simulink library "three_phase_inverter_three_level_ttype_igbt_based_model"  (R2026a)
settings: Solver=VariableStepAuto
undefined symbols (not defined in the file): DThs_init, glb_time, heatsink, igbt, Tambient
libraries: fl_lib x192, nesl_utility x108, ee_lib x24
(part 1 of 5)
settings Model: Creator=dbagn  LastModifiedBy=dbagn

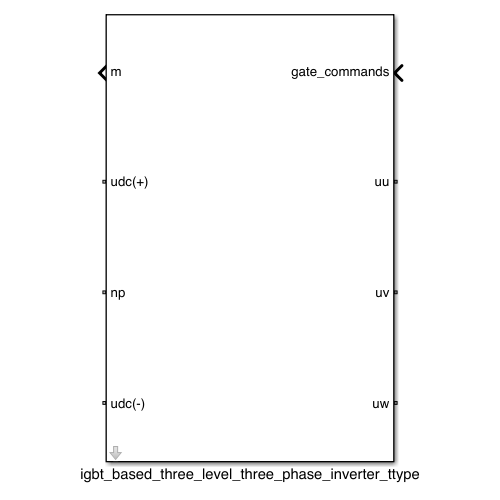
[thumbnail: Simulink's stored preview of the top-level diagram]
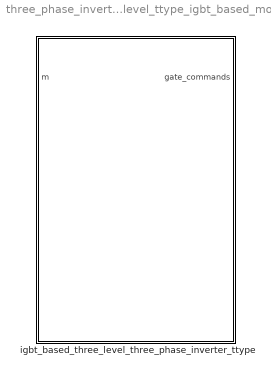
== system three_phase_inverter_three_level_ttype_igbt_based_model ==
  igbt_based_three_level_three_phase_inverter_ttype : Subsystem  mask{Vth_inv_t_m=igbt.afe.Vth, Vce_sat_inv_t_m=igbt.afe.Vce_sat, Rce_on_inv_t_m=igbt.afe.Rce_on, Eon_inv_t_m=igbt.afe.Eon, Eoff_inv_t_m=igbt.afe.Eoff, Erec_inv_t_m=igbt.afe.Erec, Ion_sw_loss_inv_t_m=igbt.afe.Ion_sw_losses, Voff_sw_loss_inv_t_m=igbt.afe.Voff_sw_losses, Vdon_diode_inv_t_m=igbt.afe.Vdon_diode, Rdon_diode_inv_t_m=igbt.afe.Rdon_diode, rth_switch_JH_inv_t_m=igbt.afe.Rth_switch_JH, rth_switch_HA_inv_t_m=heatsink.Rth_switch_HA, rth_diode_JH_inv_t_m=igbt.afe.Rth_diode_JH, rth_diode_HA_inv_t_m=heatsink.Rth_diode_HA, Csnubber_inv_t_m=igbt.afe.Csnubber, Rsnubber_inv_t_m=igbt.afe.Rsnubber, Vth_m=igbt.afe.Vth, Vce_sat_m=igbt.afe.Vce_sat, Rce_on_m=igbt.afe.Rce_on, Eon_m=igbt.afe.Eon, Eoff_m=igbt.afe.Eoff, Erec_m=igbt.afe.Erec, Ion_sw_loss_m=igbt.afe.Ion_sw_losses, Voff_sw_loss_m=igbt.afe.Voff_sw_losses, Vdon_diode_m=igbt.afe.Vdon_diode, Rdon_diode_m=igbt.afe.Rdon_diode, rth_switch_JH_m=igbt.afe.Rth_switch_JH, rth_switch_HA_m=heatsink.Rth_switch_HA, rth_diode_JH_m=igbt.afe.Rth_diode_JH, rth_diode_HA_m=heatsink.Rth_diode_HA, Csnubber_m=igbt.afe.Csnubber, Rsnubber_m=igbt.afe.Rsnubber, JunctionTermalMass_m=igbt.afe.JunctionTermalMass, mass_heatsink_m=heatsink.no_weight, specific_heat_m=heatsink.cp, Tambient_m=heatsink.Tambient, DThs_init_m=heatsink.DThs_init, tc_m=glb_time.tc}
      mask prompts: Vth_inv_t_m "Vth (V)"; Vce_sat_inv_t_m "Vce_sat (V)"; Rce_on_inv_t_m "Rce_on (Ohm)"; Eon_inv_t_m "Eon (J)"; Eoff_inv_t_m "Eoff (J)"; Erec_inv_t_m "Erec (J)"; Ion_sw_loss_inv_t_m "Ion_sw_loss (A)"; Voff_sw_loss_inv_t_m "Voff_sw_loss (V)"; Vdon_diode_inv_t_m "Vdon_diode (V)"; Rdon_diode_inv_t_m "Rdon_diode (Ohm)"; rth_switch_JH_inv_t_m "rth_switch_JH (K/W)"; rth_switch_HA_inv_t_m "rth_switch_HA  (K/W)"; rth_diode_JH_inv_t_m "rth_diode_JH (K/W)"; rth_diode_HA_inv_t_m "rth_diode_HA  (K/W)"; Csnubber_inv_t_m "Csnubber (F)"; Rsnubber_inv_t_m "Rsnubber (Ohm)"; Vth_m "Vth (V)"; Vce_sat_m "Vce_sat (V)"; Rce_on_m "Rce_on (Ohm)"; Eon_m "Eon (J)"; Eoff_m "Eoff (J)"; Erec_m "Erec (J)"; Ion_sw_loss_m "Ion_sw_loss (A)"; Voff_sw_loss_m "Voff_sw_loss (V)"; Vdon_diode_m "Vdon_diode (V)"; Rdon_diode_m "Rdon_diode (Ohm)"; rth_switch_JH_m "rth_switch_JH (K/W)"; rth_switch_HA_m "rth_switch_HA  (K/W)"; rth_diode_JH_m "rth_diode_JH (K/W)"; rth_diode_HA_m "rth_diode_HA  (K/W)"; Csnubber_m "Csnubber (F)"; Rsnubber_m "Rsnubber (Ohm)"; JunctionTermalMass_m "JunctionTermalMass (J/K)"; mass_heatsink_m "mass_heatsink (Kg)"; specific_heat_m "specific_heat (J/(K*Kg))"; Tambient_m "Tambient (Celsius)"; DThs_init_m "DThs_init (Celsius)"; tc_m "tc"
      mask DialogControl inv_t Prompt: T-IGBT
      mask DialogControl inv Prompt: IGBT
      mask DialogControl thermal Prompt: Thermal
      mask DialogControl solver Prompt: Solver

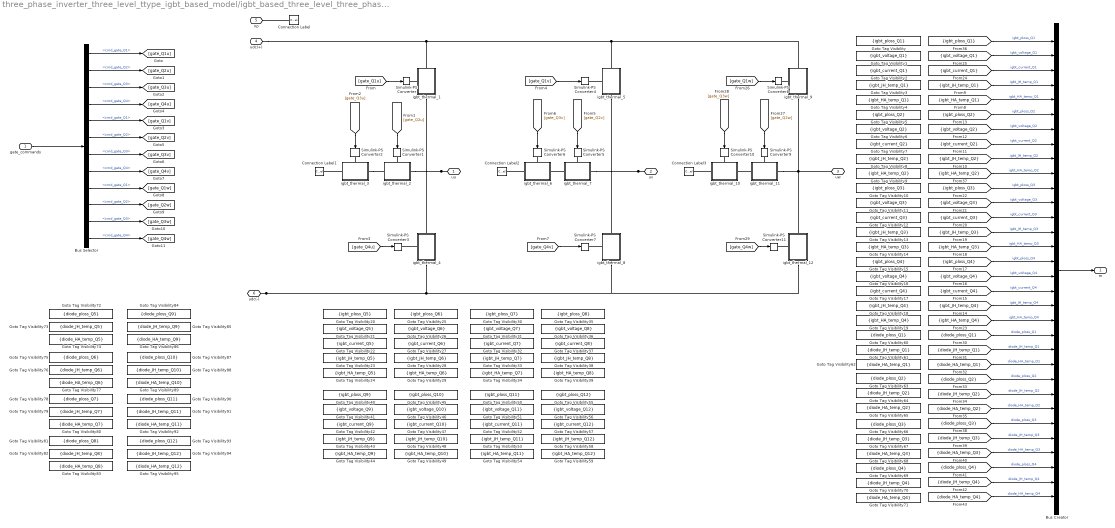
== system three_phase_inverter_three_level_ttype_igbt_based_model/igbt_based_three_level_three_phase_inverter_ttype ==
  gate_commands : Inport
  Bus Creator : BusCreator  Inputs=32
  Bus Selector : BusSelector  OutputSignals=gate_cmds_phu.cmd_gate_Q1,gate_cmds_phu.cmd_gate_Q2,gate_cmds_phu.cmd_gate_Q3,gate_cmds_phu.cmd_gate_Q4,gate_cmds_phv.cmd_gate_Q1,gate_cmds_phv.cmd_gate_Q2,gate_cmds_phv.cmd_gate_Q3,gate_cmds_phv.cmd_gate_Q4,gate_cmds_phw.cmd_gate_Q1,gate_cmds_phw.cmd_gate_Q2,gate_cmds_phw.cmd_gate_Q3,gate_cmds_phw.cmd_gate_Q4
  Connection Label{,1..3} (4 alike) : ConnectionLabel  Label=np
  Goto Tag Visibility : GotoTagVisibility  GotoTag=igbt_ploss_Q1
  Goto Tag Visibility1 : GotoTagVisibility  GotoTag=igbt_voltage_Q1
  Goto Tag Visibility10 : GotoTagVisibility  GotoTag=igbt_ploss_Q3
  Goto Tag Visibility11 : GotoTagVisibility  GotoTag=igbt_voltage_Q3
  Goto Tag Visibility12 : GotoTagVisibility  GotoTag=igbt_current_Q3
  Goto Tag Visibility13 : GotoTagVisibility  GotoTag=igbt_JH_temp_Q3
  Goto Tag Visibility14 : GotoTagVisibility  GotoTag=igbt_HA_temp_Q3
  Goto Tag Visibility15 : GotoTagVisibility  GotoTag=igbt_ploss_Q4
  Goto Tag Visibility16 : GotoTagVisibility  GotoTag=igbt_voltage_Q4
  Goto Tag Visibility17 : GotoTagVisibility  GotoTag=igbt_current_Q4
  Goto Tag Visibility18 : GotoTagVisibility  GotoTag=igbt_JH_temp_Q4
  Goto Tag Visibility19 : GotoTagVisibility  GotoTag=igbt_HA_temp_Q4
  Goto Tag Visibility2 : GotoTagVisibility  GotoTag=igbt_current_Q1
  Goto Tag Visibility20 : GotoTagVisibility  GotoTag=igbt_ploss_Q5
  Goto Tag Visibility21 : GotoTagVisibility  GotoTag=igbt_voltage_Q5
  Goto Tag Visibility22 : GotoTagVisibility  GotoTag=igbt_current_Q5
  Goto Tag Visibility23 : GotoTagVisibility  GotoTag=igbt_JH_temp_Q5
  Goto Tag Visibility24 : GotoTagVisibility  GotoTag=igbt_HA_temp_Q5
  Goto Tag Visibility25 : GotoTagVisibility  GotoTag=igbt_ploss_Q6
  Goto Tag Visibility26 : GotoTagVisibility  GotoTag=igbt_voltage_Q6
  Goto Tag Visibility27 : GotoTagVisibility  GotoTag=igbt_current_Q6
  Goto Tag Visibility28 : GotoTagVisibility  GotoTag=igbt_JH_temp_Q6
  Goto Tag Visibility29 : GotoTagVisibility  GotoTag=igbt_HA_temp_Q6
  Goto Tag Visibility3 : GotoTagVisibility  GotoTag=igbt_JH_temp_Q1
  Goto Tag Visibility30 : GotoTagVisibility  GotoTag=igbt_ploss_Q7
  Goto Tag Visibility31 : GotoTagVisibility  GotoTag=igbt_voltage_Q7
  Goto Tag Visibility32 : GotoTagVisibility  GotoTag=igbt_current_Q7
  Goto Tag Visibility33 : GotoTagVisibility  GotoTag=igbt_JH_temp_Q7
  Goto Tag Visibility34 : GotoTagVisibility  GotoTag=igbt_HA_temp_Q7
  Goto Tag Visibility35 : GotoTagVisibility  GotoTag=igbt_ploss_Q8
  Goto Tag Visibility36 : GotoTagVisibility  GotoTag=igbt_voltage_Q8
  Goto Tag Visibility37 : GotoTagVisibility  GotoTag=igbt_current_Q8
  Goto Tag Visibility38 : GotoTagVisibility  GotoTag=igbt_JH_temp_Q8
  Goto Tag Visibility39 : GotoTagVisibility  GotoTag=igbt_HA_temp_Q8
  Goto Tag Visibility4 : GotoTagVisibility  GotoTag=igbt_HA_temp_Q1
  Goto Tag Visibility40 : GotoTagVisibility  GotoTag=igbt_ploss_Q9
  Goto Tag Visibility41 : GotoTagVisibility  GotoTag=igbt_voltage_Q9
  Goto Tag Visibility42 : GotoTagVisibility  GotoTag=igbt_current_Q9
  Goto Tag Visibility43 : GotoTagVisibility  GotoTag=igbt_JH_temp_Q9
  Goto Tag Visibility44 : GotoTagVisibility  GotoTag=igbt_HA_temp_Q9
  Goto Tag Visibility45 : GotoTagVisibility  GotoTag=igbt_ploss_Q10
  Goto Tag Visibility46 : GotoTagVisibility  GotoTag=igbt_voltage_Q10
  Goto Tag Visibility47 : GotoTagVisibility  GotoTag=igbt_current_Q10
  Goto Tag Visibility48 : GotoTagVisibility  GotoTag=igbt_JH_temp_Q10
  Goto Tag Visibility49 : GotoTagVisibility  GotoTag=igbt_HA_temp_Q10
  Goto Tag Visibility5 : GotoTagVisibility  GotoTag=igbt_ploss_Q2
  Goto Tag Visibility50 : GotoTagVisibility  GotoTag=igbt_ploss_Q11
  Goto Tag Visibility51 : GotoTagVisibility  GotoTag=igbt_voltage_Q11
  Goto Tag Visibility52 : GotoTagVisibility  GotoTag=igbt_current_Q11
  Goto Tag Visibility53 : GotoTagVisibility  GotoTag=igbt_JH_temp_Q11
  Goto Tag Visibility54 : GotoTagVisibility  GotoTag=igbt_HA_temp_Q11
  Goto Tag Visibility55 : GotoTagVisibility  GotoTag=igbt_ploss_Q12
  Goto Tag Visibility56 : GotoTagVisibility  GotoTag=igbt_voltage_Q12
  Goto Tag Visibility57 : GotoTagVisibility  GotoTag=igbt_current_Q12
  Goto Tag Visibility58 : GotoTagVisibility  GotoTag=igbt_JH_temp_Q12
  Goto Tag Visibility59 : GotoTagVisibility  GotoTag=igbt_HA_temp_Q12
  Goto Tag Visibility6 : GotoTagVisibility  GotoTag=igbt_voltage_Q2
  Goto Tag Visibility60 : GotoTagVisibility  GotoTag=diode_ploss_Q1
  Goto Tag Visibility61 : GotoTagVisibility  GotoTag=diode_JH_temp_Q1
  Goto Tag Visibility62 : GotoTagVisibility  GotoTag=diode_HA_temp_Q1
  Goto Tag Visibility63 : GotoTagVisibility  GotoTag=diode_ploss_Q2
  Goto Tag Visibility64 : GotoTagVisibility  GotoTag=diode_JH_temp_Q2
  Goto Tag Visibility65 : GotoTagVisibility  GotoTag=diode_HA_temp_Q2
  Goto Tag Visibility66 : GotoTagVisibility  GotoTag=diode_ploss_Q3
  Goto Tag Visibility67 : GotoTagVisibility  GotoTag=diode_JH_temp_Q3
  Goto Tag Visibility68 : GotoTagVisibility  GotoTag=diode_HA_temp_Q3
  Goto Tag Visibility69 : GotoTagVisibility  GotoTag=diode_ploss_Q4
  Goto Tag Visibility7 : GotoTagVisibility  GotoTag=igbt_current_Q2
  Goto Tag Visibility70 : GotoTagVisibility  GotoTag=diode_JH_temp_Q4
  Goto Tag Visibility71 : GotoTagVisibility  GotoTag=diode_HA_temp_Q4
  Goto Tag Visibility72 : GotoTagVisibility  GotoTag=diode_ploss_Q5
  Goto Tag Visibility73 : GotoTagVisibility  GotoTag=diode_JH_temp_Q5
  Goto Tag Visibility74 : GotoTagVisibility  GotoTag=diode_HA_temp_Q5
  Goto Tag Visibility75 : GotoTagVisibility  GotoTag=diode_ploss_Q6
  Goto Tag Visibility76 : GotoTagVisibility  GotoTag=diode_JH_temp_Q6
  Goto Tag Visibility77 : GotoTagVisibility  GotoTag=diode_HA_temp_Q6
  Goto Tag Visibility78 : GotoTagVisibility  GotoTag=diode_ploss_Q7
  Goto Tag Visibility79 : GotoTagVisibility  GotoTag=diode_JH_temp_Q7
  Goto Tag Visibility8 : GotoTagVisibility  GotoTag=igbt_JH_temp_Q2
  Goto Tag Visibility80 : GotoTagVisibility  GotoTag=diode_HA_temp_Q7
  Goto Tag Visibility81 : GotoTagVisibility  GotoTag=diode_ploss_Q8
  Goto Tag Visibility82 : GotoTagVisibility  GotoTag=diode_JH_temp_Q8
  Goto Tag Visibility83 : GotoTagVisibility  GotoTag=diode_HA_temp_Q8
  Goto Tag Visibility84 : GotoTagVisibility  GotoTag=diode_ploss_Q9
  Goto Tag Visibility85 : GotoTagVisibility  GotoTag=diode_JH_temp_Q9
  Goto Tag Visibility86 : GotoTagVisibility  GotoTag=diode_HA_temp_Q9
  Goto Tag Visibility87 : GotoTagVisibility  GotoTag=diode_ploss_Q10
  Goto Tag Visibility88 : GotoTagVisibility  GotoTag=diode_JH_temp_Q10
  Goto Tag Visibility89 : GotoTagVisibility  GotoTag=diode_HA_temp_Q10
  Goto Tag Visibility9 : GotoTagVisibility  GotoTag=igbt_HA_temp_Q2
  Goto Tag Visibility90 : GotoTagVisibility  GotoTag=diode_ploss_Q11
  Goto Tag Visibility91 : GotoTagVisibility  GotoTag=diode_JH_temp_Q11
  Goto Tag Visibility92 : GotoTagVisibility  GotoTag=diode_HA_temp_Q11
  Goto Tag Visibility93 : GotoTagVisibility  GotoTag=diode_ploss_Q12
  Goto Tag Visibility94 : GotoTagVisibility  GotoTag=diode_JH_temp_Q12
  Goto Tag Visibility95 : GotoTagVisibility  GotoTag=diode_HA_temp_Q12
  Simulink-PS Converter{,1..11} (12 alike) : nesl_utility/Simulink-PS Converter  PhysicalDomain=network_engine_domain  SubClassName=ps_input  LeftPortType=input  RightPortType=output  PseudoPeriodic=off  Frequencies=[]  NoiseDistribution=none  NoiseParameters=[]  Unit=1  AffineConversion=on  FilteringAndDerivatives=provide  SimscapeFilterOrder=1  InputFilterTimeConstant=0.001  UdotUserProvided=0
  igbt_thermal_1 : Subsystem
      settings: PortSchema="{\"entries\":[{\"content\":{\"sides\":[{\"content\":{\"connectorIds\":[\"LConn1\"]},\"type\":\"ConnectorPlacement.EquallySpacedRectSide\",\"uuid\":\"9277da8d-d460-43e6-8478-dd662f15d226\"},{\"content\":{\"connectorIds\":[],\"side\":\"RIGHT\"},\"type\":\"ConnectorPlacement.EquallySpacedRectSide\",\"uuid\":\"a7ece396-f1d9-4f4f-a05b-db1fc65d6e1d\"},{\"content\":{\"connectorIds\":[\"LConn2\"],\"side\":\"TOP\"},\"type\":\"ConnectorPlacement.EquallySpacedRectSide\",\"uuid\":\"fdd70777-e9cf-4317-afb6-cae87f75d5b0\"},{\"content\":{\"connectorIds\":[\"RConn1\"],\"side\":\"BOTTOM\"},\"type\":\"ConnectorPlacement.EquallySpacedRectSide\",\"uuid\":\"2353ed68-b1a1-4775-9ca9-31e268d5443b\"}]},\"type\":\"ConnectorPlacement.EquallySpacedConnector\",\"uuid\":\"d5479f4c-4e65-4791-adcb-73df11f88590\"}],\"packageUris\":[\"http://schema.mathworks.com/mf0/Connector/R2020b\"],\"version\":\"1.0\"}"
  igbt_thermal_10 : Subsystem
      settings: PortSchema="{\"entries\":[{\"content\":{\"sides\":[{\"content\":{\"connectorIds\":[\"LConn1\"]},\"type\":\"ConnectorPlacement.EquallySpacedRectSide\",\"uuid\":\"9277da8d-d460-43e6-8478-dd662f15d226\"},{\"content\":{\"connectorIds\":[],\"side\":\"RIGHT\"},\"type\":\"ConnectorPlacement.EquallySpacedRectSide\",\"uuid\":\"a7ece396-f1d9-4f4f-a05b-db1fc65d6e1d\"},{\"content\":{\"connectorIds\":[\"LConn2\"],\"side\":\"TOP\"},\"type\":\"ConnectorPlacement.EquallySpacedRectSide\",\"uuid\":\"fdd70777-e9cf-4317-afb6-cae87f75d5b0\"},{\"content\":{\"connectorIds\":[\"RConn1\"],\"side\":\"BOTTOM\"},\"type\":\"ConnectorPlacement.EquallySpacedRectSide\",\"uuid\":\"2353ed68-b1a1-4775-9ca9-31e268d5443b\"}]},\"type\":\"ConnectorPlacement.EquallySpacedConnector\",\"uuid\":\"d5479f4c-4e65-4791-adcb-73df11f88590\"}],\"packageUris\":[\"http://schema.mathworks.com/mf0/Connector/R2020b\"],\"version\":\"1.0\"}"
  igbt_thermal_11 : Subsystem
      settings: PortSchema="{\"entries\":[{\"content\":{\"sides\":[{\"content\":{\"connectorIds\":[\"LConn1\"]},\"type\":\"ConnectorPlacement.EquallySpacedRectSide\",\"uuid\":\"9277da8d-d460-43e6-8478-dd662f15d226\"},{\"content\":{\"connectorIds\":[],\"side\":\"RIGHT\"},\"type\":\"ConnectorPlacement.EquallySpacedRectSide\",\"uuid\":\"a7ece396-f1d9-4f4f-a05b-db1fc65d6e1d\"},{\"content\":{\"connectorIds\":[\"LConn2\"],\"side\":\"TOP\"},\"type\":\"ConnectorPlacement.EquallySpacedRectSide\",\"uuid\":\"fdd70777-e9cf-4317-afb6-cae87f75d5b0\"},{\"content\":{\"connectorIds\":[\"RConn1\"],\"side\":\"BOTTOM\"},\"type\":\"ConnectorPlacement.EquallySpacedRectSide\",\"uuid\":\"2353ed68-b1a1-4775-9ca9-31e268d5443b\"}]},\"type\":\"ConnectorPlacement.EquallySpacedConnector\",\"uuid\":\"d5479f4c-4e65-4791-adcb-73df11f88590\"}],\"packageUris\":[\"http://schema.mathworks.com/mf0/Connector/R2020b\"],\"version\":\"1.0\"}"
  igbt_thermal_12 : Subsystem
      settings: PortSchema="{\"entries\":[{\"content\":{\"sides\":[{\"content\":{\"connectorIds\":[\"LConn1\"]},\"type\":\"ConnectorPlacement.EquallySpacedRectSide\",\"uuid\":\"9277da8d-d460-43e6-8478-dd662f15d226\"},{\"content\":{\"connectorIds\":[],\"side\":\"RIGHT\"},\"type\":\"ConnectorPlacement.EquallySpacedRectSide\",\"uuid\":\"a7ece396-f1d9-4f4f-a05b-db1fc65d6e1d\"},{\"content\":{\"connectorIds\":[\"LConn2\"],\"side\":\"TOP\"},\"type\":\"ConnectorPlacement.EquallySpacedRectSide\",\"uuid\":\"fdd70777-e9cf-4317-afb6-cae87f75d5b0\"},{\"content\":{\"connectorIds\":[\"RConn1\"],\"side\":\"BOTTOM\"},\"type\":\"ConnectorPlacement.EquallySpacedRectSide\",\"uuid\":\"2353ed68-b1a1-4775-9ca9-31e268d5443b\"}]},\"type\":\"ConnectorPlacement.EquallySpacedConnector\",\"uuid\":\"d5479f4c-4e65-4791-adcb-73df11f88590\"}],\"packageUris\":[\"http://schema.mathworks.com/mf0/Connector/R2020b\"],\"version\":\"1.0\"}"
  igbt_thermal_2 : Subsystem
      settings: PortSchema="{\"entries\":[{\"content\":{\"sides\":[{\"content\":{\"connectorIds\":[\"LConn1\"]},\"type\":\"ConnectorPlacement.EquallySpacedRectSide\",\"uuid\":\"9277da8d-d460-43e6-8478-dd662f15d226\"},{\"content\":{\"connectorIds\":[],\"side\":\"RIGHT\"},\"type\":\"ConnectorPlacement.EquallySpacedRectSide\",\"uuid\":\"a7ece396-f1d9-4f4f-a05b-db1fc65d6e1d\"},{\"content\":{\"connectorIds\":[\"LConn2\"],\"side\":\"TOP\"},\"type\":\"ConnectorPlacement.EquallySpacedRectSide\",\"uuid\":\"fdd70777-e9cf-4317-afb6-cae87f75d5b0\"},{\"content\":{\"connectorIds\":[\"RConn1\"],\"side\":\"BOTTOM\"},\"type\":\"ConnectorPlacement.EquallySpacedRectSide\",\"uuid\":\"2353ed68-b1a1-4775-9ca9-31e268d5443b\"}]},\"type\":\"ConnectorPlacement.EquallySpacedConnector\",\"uuid\":\"d5479f4c-4e65-4791-adcb-73df11f88590\"}],\"packageUris\":[\"http://schema.mathworks.com/mf0/Connector/R2020b\"],\"version\":\"1.0\"}"
  igbt_thermal_3 : Subsystem
      settings: PortSchema="{\"entries\":[{\"content\":{\"sides\":[{\"content\":{\"connectorIds\":[\"LConn1\"]},\"type\":\"ConnectorPlacement.EquallySpacedRectSide\",\"uuid\":\"9277da8d-d460-43e6-8478-dd662f15d226\"},{\"content\":{\"side\":\"RIGHT\"},\"type\":\"ConnectorPlacement.EquallySpacedRectSide\",\"uuid\":\"a7ece396-f1d9-4f4f-a05b-db1fc65d6e1d\"},{\"content\":{\"connectorIds\":[\"LConn2\"],\"side\":\"TOP\"},\"type\":\"ConnectorPlacement.EquallySpacedRectSide\",\"uuid\":\"fdd70777-e9cf-4317-afb6-cae87f75d5b0\"},{\"content\":{\"connectorIds\":[\"RConn1\"],\"side\":\"BOTTOM\"},\"type\":\"ConnectorPlacement.EquallySpacedRectSide\",\"uuid\":\"2353ed68-b1a1-4775-9ca9-31e268d5443b\"}]},\"type\":\"ConnectorPlacement.EquallySpacedConnector\",\"uuid\":\"d5479f4c-4e65-4791-adcb-73df11f88590\"}],\"packageUris\":[\"http://schema.mathworks.com/mf0/Connector/R2020b\"],\"version\":\"1.0\"}"
  igbt_thermal_4 : Subsystem
      settings: PortSchema="{\"entries\":[{\"content\":{\"sides\":[{\"content\":{\"connectorIds\":[\"LConn1\"]},\"type\":\"ConnectorPlacement.EquallySpacedRectSide\",\"uuid\":\"9277da8d-d460-43e6-8478-dd662f15d226\"},{\"content\":{\"connectorIds\":[],\"side\":\"RIGHT\"},\"type\":\"ConnectorPlacement.EquallySpacedRectSide\",\"uuid\":\"a7ece396-f1d9-4f4f-a05b-db1fc65d6e1d\"},{\"content\":{\"connectorIds\":[\"LConn2\"],\"side\":\"TOP\"},\"type\":\"ConnectorPlacement.EquallySpacedRectSide\",\"uuid\":\"fdd70777-e9cf-4317-afb6-cae87f75d5b0\"},{\"content\":{\"connectorIds\":[\"RConn1\"],\"side\":\"BOTTOM\"},\"type\":\"ConnectorPlacement.EquallySpacedRectSide\",\"uuid\":\"2353ed68-b1a1-4775-9ca9-31e268d5443b\"}]},\"type\":\"ConnectorPlacement.EquallySpacedConnector\",\"uuid\":\"d5479f4c-4e65-4791-adcb-73df11f88590\"}],\"packageUris\":[\"http://schema.mathworks.com/mf0/Connector/R2020b\"],\"version\":\"1.0\"}"
  igbt_thermal_5 : Subsystem
      settings: PortSchema="{\"entries\":[{\"content\":{\"sides\":[{\"content\":{\"connectorIds\":[\"LConn1\"]},\"type\":\"ConnectorPlacement.EquallySpacedRectSide\",\"uuid\":\"9277da8d-d460-43e6-8478-dd662f15d226\"},{\"content\":{\"connectorIds\":[],\"side\":\"RIGHT\"},\"type\":\"ConnectorPlacement.EquallySpacedRectSide\",\"uuid\":\"a7ece396-f1d9-4f4f-a05b-db1fc65d6e1d\"},{\"content\":{\"connectorIds\":[\"LConn2\"],\"side\":\"TOP\"},\"type\":\"ConnectorPlacement.EquallySpacedRectSide\",\"uuid\":\"fdd70777-e9cf-4317-afb6-cae87f75d5b0\"},{\"content\":{\"connectorIds\":[\"RConn1\"],\"side\":\"BOTTOM\"},\"type\":\"ConnectorPlacement.EquallySpacedRectSide\",\"uuid\":\"2353ed68-b1a1-4775-9ca9-31e268d5443b\"}]},\"type\":\"ConnectorPlacement.EquallySpacedConnector\",\"uuid\":\"d5479f4c-4e65-4791-adcb-73df11f88590\"}],\"packageUris\":[\"http://schema.mathworks.com/mf0/Connector/R2020b\"],\"version\":\"1.0\"}"
  igbt_thermal_6 : Subsystem
      settings: PortSchema="{\"entries\":[{\"content\":{\"sides\":[{\"content\":{\"connectorIds\":[\"LConn1\"]},\"type\":\"ConnectorPlacement.EquallySpacedRectSide\",\"uuid\":\"9277da8d-d460-43e6-8478-dd662f15d226\"},{\"content\":{\"side\":\"RIGHT\"},\"type\":\"ConnectorPlacement.EquallySpacedRectSide\",\"uuid\":\"a7ece396-f1d9-4f4f-a05b-db1fc65d6e1d\"},{\"content\":{\"connectorIds\":[\"LConn2\"],\"side\":\"TOP\"},\"type\":\"ConnectorPlacement.EquallySpacedRectSide\",\"uuid\":\"fdd70777-e9cf-4317-afb6-cae87f75d5b0\"},{\"content\":{\"connectorIds\":[\"RConn1\"],\"side\":\"BOTTOM\"},\"type\":\"ConnectorPlacement.EquallySpacedRectSide\",\"uuid\":\"2353ed68-b1a1-4775-9ca9-31e268d5443b\"}]},\"type\":\"ConnectorPlacement.EquallySpacedConnector\",\"uuid\":\"d5479f4c-4e65-4791-adcb-73df11f88590\"}],\"packageUris\":[\"http://schema.mathworks.com/mf0/Connector/R2020b\"],\"version\":\"1.0\"}"
  igbt_thermal_7 : Subsystem
      settings: PortSchema="{\"entries\":[{\"content\":{\"sides\":[{\"content\":{\"connectorIds\":[\"LConn1\"]},\"type\":\"ConnectorPlacement.EquallySpacedRectSide\",\"uuid\":\"9277da8d-d460-43e6-8478-dd662f15d226\"},{\"content\":{\"connectorIds\":[],\"side\":\"RIGHT\"},\"type\":\"ConnectorPlacement.EquallySpacedRectSide\",\"uuid\":\"a7ece396-f1d9-4f4f-a05b-db1fc65d6e1d\"},{\"content\":{\"connectorIds\":[\"LConn2\"],\"side\":\"TOP\"},\"type\":\"ConnectorPlacement.EquallySpacedRectSide\",\"uuid\":\"fdd70777-e9cf-4317-afb6-cae87f75d5b0\"},{\"content\":{\"connectorIds\":[\"RConn1\"],\"side\":\"BOTTOM\"},\"type\":\"ConnectorPlacement.EquallySpacedRectSide\",\"uuid\":\"2353ed68-b1a1-4775-9ca9-31e268d5443b\"}]},\"type\":\"ConnectorPlacement.EquallySpacedConnector\",\"uuid\":\"d5479f4c-4e65-4791-adcb-73df11f88590\"}],\"packageUris\":[\"http://schema.mathworks.com/mf0/Connector/R2020b\"],\"version\":\"1.0\"}"
  igbt_thermal_8 : Subsystem
      settings: PortSchema="{\"entries\":[{\"content\":{\"sides\":[{\"content\":{\"connectorIds\":[\"LConn1\"]},\"type\":\"ConnectorPlacement.EquallySpacedRectSide\",\"uuid\":\"9277da8d-d460-43e6-8478-dd662f15d226\"},{\"content\":{\"connectorIds\":[],\"side\":\"RIGHT\"},\"type\":\"ConnectorPlacement.EquallySpacedRectSide\",\"uuid\":\"a7ece396-f1d9-4f4f-a05b-db1fc65d6e1d\"},{\"content\":{\"connectorIds\":[\"LConn2\"],\"side\":\"TOP\"},\"type\":\"ConnectorPlacement.EquallySpacedRectSide\",\"uuid\":\"fdd70777-e9cf-4317-afb6-cae87f75d5b0\"},{\"content\":{\"connectorIds\":[\"RConn1\"],\"side\":\"BOTTOM\"},\"type\":\"ConnectorPlacement.EquallySpacedRectSide\",\"uuid\":\"2353ed68-b1a1-4775-9ca9-31e268d5443b\"}]},\"type\":\"ConnectorPlacement.EquallySpacedConnector\",\"uuid\":\"d5479f4c-4e65-4791-adcb-73df11f88590\"}],\"packageUris\":[\"http://schema.mathworks.com/mf0/Connector/R2020b\"],\"version\":\"1.0\"}"
  igbt_thermal_9 : Subsystem
      settings: PortSchema="{\"entries\":[{\"content\":{\"sides\":[{\"content\":{\"connectorIds\":[\"LConn1\"]},\"type\":\"ConnectorPlacement.EquallySpacedRectSide\",\"uuid\":\"9277da8d-d460-43e6-8478-dd662f15d226\"},{\"content\":{\"connectorIds\":[],\"side\":\"RIGHT\"},\"type\":\"ConnectorPlacement.EquallySpacedRectSide\",\"uuid\":\"a7ece396-f1d9-4f4f-a05b-db1fc65d6e1d\"},{\"content\":{\"connectorIds\":[\"LConn2\"],\"side\":\"TOP\"},\"type\":\"ConnectorPlacement.EquallySpacedRectSide\",\"uuid\":\"fdd70777-e9cf-4317-afb6-cae87f75d5b0\"},{\"content\":{\"connectorIds\":[\"RConn1\"],\"side\":\"BOTTOM\"},\"type\":\"ConnectorPlacement.EquallySpacedRectSide\",\"uuid\":\"2353ed68-b1a1-4775-9ca9-31e268d5443b\"}]},\"type\":\"ConnectorPlacement.EquallySpacedConnector\",\"uuid\":\"d5479f4c-4e65-4791-adcb-73df11f88590\"}],\"packageUris\":[\"http://schema.mathworks.com/mf0/Connector/R2020b\"],\"version\":\"1.0\"}"
  uu : PMIOPort  Side=Left
  uv : PMIOPort  Port=2  Side=Left
  uw : PMIOPort  Port=3  Side=Left
  udc(+) : PMIOPort  Port=4  Side=Right
  np : PMIOPort  Port=5  Side=Right
  udc(-) : PMIOPort  Port=6  Side=Right
  m : Outport
  wires:
  [gate_Q4u] -> Simulink-PS Converter3/1
  [gate_Q3u] -> Simulink-PS Converter2/1
  [gate_Q2u] -> Simulink-PS Converter1/1
  [gate_Q1u] -> Simulink-PS Converter/1
  [gate_Q1v] -> Simulink-PS Converter4/1
  [gate_Q2v] -> Simulink-PS Converter5/1
  [gate_Q3v] -> Simulink-PS Converter6/1
  [gate_Q4v] -> Simulink-PS Converter7/1
  gate_commands/1 -> Bus Selector/1
  [igbt_voltage_Q1] -> Bus Creator/2  "igbt_voltage_Q1"
  [igbt_current_Q4] -> Bus Creator/18  "igbt_current_Q4"
  [igbt_voltage_Q2] -> Bus Creator/7  "igbt_voltage_Q2"
  [igbt_ploss_Q2] -> Bus Creator/6  "igbt_ploss_Q2"
  Bus Creator/1 -> m/1
  [igbt_ploss_Q3] -> Bus Creator/11  "igbt_ploss_Q3"
  [igbt_HA_temp_Q1] -> Bus Creator/5  "igbt_HA_temp_Q1"
  [igbt_ploss_Q1] -> Bus Creator/1  "igbt_ploss_Q1"
  [igbt_voltage_Q4] -> Bus Creator/17  "igbt_voltage_Q4"
  [igbt_ploss_Q4] -> Bus Creator/16  "igbt_ploss_Q4"
  [igbt_JH_temp_Q4] -> Bus Creator/19  "igbt_JH_temp_Q4"
  [igbt_voltage_Q3] -> Bus Creator/12  "igbt_voltage_Q3"
  [igbt_current_Q1] -> Bus Creator/3  "igbt_current_Q1"
  [igbt_HA_temp_Q4] -> Bus Creator/20  "igbt_HA_temp_Q4"
  [igbt_JH_temp_Q3] -> Bus Creator/14  "igbt_JH_temp_Q3"
  [igbt_current_Q2] -> Bus Creator/8  "igbt_current_Q2"
  [igbt_HA_temp_Q2] -> Bus Creator/10  "igbt_HA_temp_Q2"
  [igbt_JH_temp_Q2] -> Bus Creator/9  "igbt_JH_temp_Q2"
  [igbt_JH_temp_Q1] -> Bus Creator/4  "igbt_JH_temp_Q1"
  [igbt_current_Q3] -> Bus Creator/13  "igbt_current_Q3"
  [igbt_HA_temp_Q3] -> Bus Creator/15  "igbt_HA_temp_Q3"
  [gate_Q4w] -> Simulink-PS Converter11/1
  [gate_Q3w] -> Simulink-PS Converter10/1
  [gate_Q2w] -> Simulink-PS Converter9/1
  [gate_Q1w] -> Simulink-PS Converter8/1
  [diode_ploss_Q1] -> Bus Creator/21  "diode_ploss_Q1"
  [diode_JH_temp_Q1] -> Bus Creator/22  "diode_JH_temp_Q1"
  [diode_HA_temp_Q1] -> Bus Creator/23  "diode_HA_temp_Q1"
  [diode_ploss_Q2] -> Bus Creator/24  "diode_ploss_Q2"
  [diode_JH_temp_Q2] -> Bus Creator/25  "diode_JH_temp_Q2"
  [diode_HA_temp_Q2] -> Bus Creator/26  "diode_HA_temp_Q2"
  [diode_ploss_Q3] -> Bus Creator/27  "diode_ploss_Q3"
  [diode_JH_temp_Q3] -> Bus Creator/28  "diode_JH_temp_Q3"
  [diode_HA_temp_Q3] -> Bus Creator/29  "diode_HA_temp_Q3"
  [diode_HA_temp_Q4] -> Bus Creator/32  "diode_HA_temp_Q4"
  [diode_JH_temp_Q4] -> Bus Creator/31  "diode_JH_temp_Q4"
  [diode_ploss_Q4] -> Bus Creator/30  "diode_ploss_Q4"
  Bus Selector/1 -> [gate_Q1u]  "<cmd_gate_Q1>"
  Bus Selector/2 -> [gate_Q2u]  "<cmd_gate_Q2>"
  Bus Selector/3 -> [gate_Q3u]  "<cmd_gate_Q3>"
  Bus Selector/9 -> [gate_Q1w]  "<cmd_gate_Q1>"
  Bus Selector/4 -> [gate_Q4u]  "<cmd_gate_Q4>"
  Bus Selector/5 -> [gate_Q1v]  "<cmd_gate_Q1>"
  Bus Selector/6 -> [gate_Q2v]  "<cmd_gate_Q2>"
  Bus Selector/7 -> [gate_Q3v]  "<cmd_gate_Q3>"
  Bus Selector/8 -> [gate_Q4v]  "<cmd_gate_Q4>"
  Bus Selector/10 -> [gate_Q2w]  "<cmd_gate_Q2>"
  Bus Selector/12 -> [gate_Q4w]  "<cmd_gate_Q4>"
  Bus Selector/11 -> [gate_Q3w]  "<cmd_gate_Q3>"
  connections:
  udc(+)/RConn1 -- igbt_thermal_1/LConn2 -- igbt_thermal_5/LConn2 -- igbt_thermal_9/LConn2
  igbt_thermal_4/LConn1 -- Simulink-PS Converter3/RConn1
  igbt_thermal_3/LConn1 -- Simulink-PS Converter2/RConn1
  igbt_thermal_2/LConn1 -- Simulink-PS Converter1/RConn1
  igbt_thermal_1/LConn1 -- Simulink-PS Converter/RConn1
  igbt_thermal_7/LConn1 -- Simulink-PS Converter5/RConn1
  igbt_thermal_6/LConn1 -- Simulink-PS Converter6/RConn1
  igbt_thermal_8/LConn1 -- Simulink-PS Converter7/RConn1
  uu/RConn1 -- igbt_thermal_2/RConn1 -- igbt_thermal_4/LConn2 -- igbt_thermal_1/RConn1
  udc(-)/RConn1 -- igbt_thermal_12/RConn1 -- igbt_thermal_8/RConn1 -- igbt_thermal_4/RConn1
  uv/RConn1 -- igbt_thermal_5/RConn1 -- igbt_thermal_8/LConn2 -- igbt_thermal_7/RConn1
  igbt_thermal_7/LConn2 -- igbt_thermal_6/LConn2
  Connection Label/LConn1 -- np/RConn1
  igbt_thermal_3/RConn1 -- Connection Label1/LConn1
  igbt_thermal_6/RConn1 -- Connection Label2/LConn1
  igbt_thermal_9/RConn1 -- igbt_thermal_12/LConn2 -- igbt_thermal_11/RConn1 -- uw/RConn1
  igbt_thermal_9/LConn1 -- Simulink-PS Converter8/RConn1
  igbt_thermal_3/LConn2 -- igbt_thermal_2/LConn2
  igbt_thermal_12/LConn1 -- Simulink-PS Converter11/RConn1
  igbt_thermal_10/LConn1 -- Simulink-PS Converter10/RConn1
  igbt_thermal_10/RConn1 -- Connection Label3/LConn1
  igbt_thermal_11/LConn1 -- Simulink-PS Converter9/RConn1
  igbt_thermal_11/LConn2 -- igbt_thermal_10/LConn2
  igbt_thermal_5/LConn1 -- Simulink-PS Converter4/RConn1

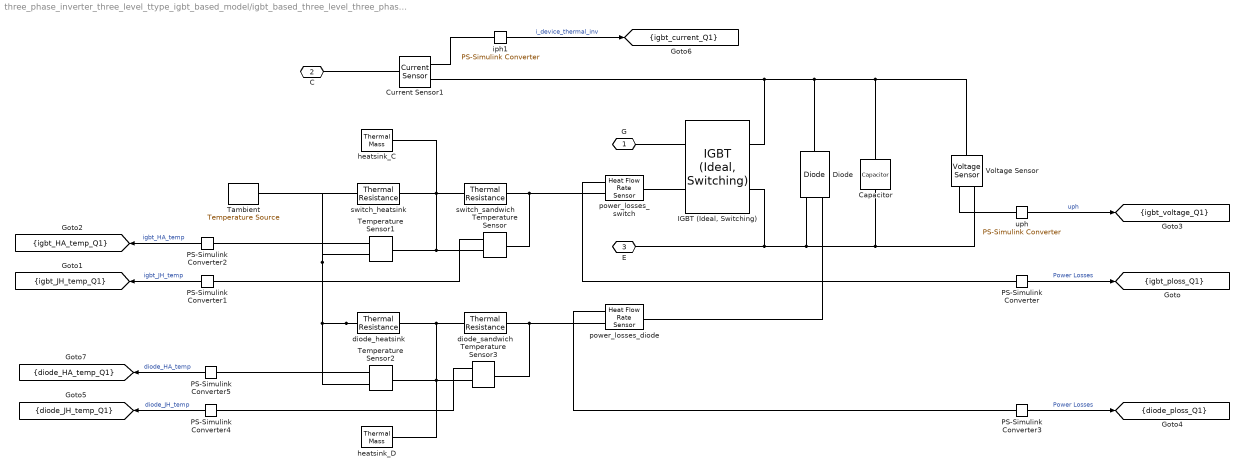
== system three_phase_inverter_three_level_ttype_igbt_based_model/igbt_based_three_level_three_phase_inverter_ttype/igbt_thermal_1 ==
  Capacitor : fl_lib/Electrical/Electrical Elements/Capacitor  c=Csnubber_m F  r=Rsnubber_m Ohm  g=0 1/Ohm  i_specify=off  i_priority=None  i=0 A  i_nominal_specify=off  i_nominal_value=1  i_nominal_unit=A  v_specify=off  v_priority=None  v=0 V  v_nominal_specify=off  v_nominal_value=1  v_nominal_unit=V  vc_specify=off  vc_priority=High  vc=0 V  vc_nominal_specify=off  vc_nominal_value=1  vc_nominal_unit=V
  Current Sensor1 : fl_lib/Electrical/Electrical Sensors/Current Sensor
  Diode : ee_lib/Semiconductors & Converters/Diode  ModelType=ee.enum.diode.modelType.pwl  TableType=ee.enum.diode.tableType.IfMat  IfMat=[.07, .12, .19, 1.75, 4.24, 7.32, 11.2; .16, .3, .72, 2.14, 5.02, 8.35, 13.12] A  VfMat=[.9, 1.15, 1.25, 1.5, 1.75, 2.17, 2.6, 2.85; .58, .68, .75, 1.1, 1.38, 1.77, 2.27, 2.7] V  TjVec=[25, 125] degC  VfVec=[.5, .7, .9, 1.3, 1.7, 2.1, 2.5] V  IfVec=[.1, .2, .5, 1, 2, 4, 7, 10] A  IrMat=[1e-06, 2e-06, 5e-06, 1e-05, 2.5e-05, 5e-05, .0001; 2e-06, 5e-06, 1e-05, 4e-05, 8e-05, .0002, .0005] A  VrMat=[10, 100, 200, 250, 300, 325, 350; 10, 70, 160, 220, 270, 300, 320] V  VrVec=[10, 20, 40, 50, 70, 80, 100] V  IrVec=[1e-06, 2e-06, 5e-06, 1e-05, 2e-05, 5e-05, .0001] A  Vf=Vdon_diode_m V  Ron=Rdon_diode_m Ohm  Goff=1e-8 S  prmExp=ee.enum.diode.expParam.useTwo  I12=[.0137, .545] A  V12=[.6, .7] V  RS=0 Ohm  Tmeas=298.15 K  IS=1e-12 A  ec=1  I1=0.0137 A  V1=0.6 V  N_series=1  N_parallel=1  ZenerEnable=false  Rz=0.3 Ohm  BV=inf V  C_param=ee.enum.diode.capParam.fixed  CJ=0 pF  CJ0=5 pF  Vvec=[.1, 10, 100] V  Cvec=[3.5, 1, .4] pF  VJ=1 V  Mgrad=0.5  FC=0.5  Q_param=ee.enum.diode.recoveryParam.off  iRM=-7.15 A  iF=4 A  didt=-750 A/us  trr_factor=3  trr=115 ns  Qrr=150 nA*s  Vr=-600 V  Ls=150 nH  Erec=0.03 J  TT=50 ns  tau=100 ns  T_param=ee.enum.diode.temperatureParam.off  Tdevice=298.15 K  I1_T2=0.245 A  V1_T2=0.5 V  IS_T2=1.25e-7 A  Tmeas2=125 degC  XTI_param=ee.enum.diode.xtiParam.pn  XTI=3  EG_param=ee.enum.diode.egapParam.material_si  EG=1.11 eV  dBVdT=0 V/K  enable_fault_input=simscape.enum.onoff.off  i_specify=off  i_priority=None  i=0 A  i_nominal_specify=off  i_nominal_value=1  i_nominal_unit=A  v_specify=off  v_priority=None  v=0 V  v_nominal_specify=off  v_nominal_value=1  v_nominal_unit=V  v_capacitor_specify=off  v_capacitor_priority=None  v_capacitor=0 V  v_capacitor_nominal_specify=off  v_capacitor_nominal_value=1  v_capacitor_nominal_unit=V  Qj_specify=off  Qj_priority=High  Qj=0 C  Qj_nominal_specify=off  Qj_nominal_value=1  Qj_nominal_unit=C  i_diode_specify=off  i_diode_priority=None  i_diode=0 A  i_diode_nominal_specify=off  i_diode_nominal_value=1  i_diode_nominal_unit=A  v_diode_specify=off  v_diode_priority=None  v_diode=0 V  v_diode_nominal_specify=off  v_diode_nominal_value=1  v_diode_nominal_unit=V  i_capacitor_specify=off  i_capacitor_priority=None  i_capacitor=0 A  i_capacitor_nominal_specify=off  i_capacitor_nominal_value=1  i_capacitor_nominal_unit=A  fidelity_level=ee.enum.diode.fidelity.idealSwitch  rec_loss_model=ee.enum.diode.reverseRecoveryModel.fixed  ErecVal=Erec_m J  scaleWithIandV=true  ErecMat=zeros(2, 3) J  ErecMat3D=zeros(2, 3, 2) J  TjrecVec=[298.15, 398.15] K  IfrecVec=[.1, 1, 10] A  IrecVal=Ion_sw_loss_m A  VrecVal=Voff_sw_loss_m V  VrecVec=[0, 100] V  tFilter=tc_m s  thermal_network_parameterization=ee.enum.thermalNetworkTopology.external  Rth=[0, 10] K/W  Rth_Cauer=[1, 3, 10] K/W  Rth_Foster=[.08, .14, .22, .16] K/W  thermal_mass_parameterization=ee.enum.thermalNetwork.timeconstant  thermal_mass=[0, 1] J/K  thermal_mass_Cauer=[.1, .3, 1] J/K  thermal_mass_Foster=[.001, .005, .05, .5] J/K  thermal_time_constant=[0, 10] s  thermal_time_constant_Cauer=[1, 3, 10] s  thermal_time_constant_Foster=[7e-05, .0007, .01, .08] s  thermal_mass_initial_temperatures=[25, 25] degC  thermal_mass_initial_temperatures_Cauer=[25, 25, 25] degC  junction_thermal_mass=JunctionTermalMass_m J/K  Tvec_initial_Foster=[25, 25, 25, 25] degC  no_thermal_network=0  junction_temperature_specify=off  junction_temperature_priority=None  junction_temperature=25 degC  junction_temperature_nominal_specify=off  junction_temperature_nominal_value=1  junction_temperature_nominal_unit=degC
  "IGBT (Ideal, Switching)" : ee_lib/Semiconductors & Converters/IGBT (Ideal, Switching)  port_option=ee.enum.controlport.ps  Vf=Vce_sat_m V  Ron=Rce_on_m Ohm  Goff=1e-5 1/Ohm  Vth=Vth_m V  diode_param=ee.enum.semiconductors.protectionDiode.external  diode_Vf=Vdon_diode_m V  diode_Ron=Rdon_diode_m Ohm  diode_Goff=1e-5 1/Ohm  diode_C=50e-9 F  diode_iRM=-235 A  diode_iF=300 A  diode_idot=-50 A/us  diode_trr_param=ee.enum.converters.diodeReverseParam.trr_factor  diode_trr_factor=3  diode_trr=15 us  diode_Qrr=1500 s*uA  ice_specify=off  ice_priority=None  ice=0 A  ice_nominal_specify=off  ice_nominal_value=1  ice_nominal_unit=A  vce_specify=off  vce_priority=None  vce=0 V  vce_nominal_specify=off  vce_nominal_value=1  vce_nominal_unit=V  vge_specify=off  vge_priority=None  vge=0 V  vge_nominal_specify=off  vge_nominal_value=1  vge_nominal_unit=V  thermal_loss_option=ee.enum.converters.thermalLossOption.constantvalues  Von_data=[0, .1, .6, .8, 1, 1.3, 1.6, 2, 2.4; 0, .1, .7, 1, 1.2, 1.5, 1.9, 2.4, 2.8] V  Tj=[298.15, 398.15] K  Iout_data=[0, .1, 1, 5, 10, 20, 40, 70, 100] A  tabulateWithVce=false  Eon_data=[0, .0024, .024, .12, .2, .48, 1.04, 2.16, 3.24; 0, .003, .03, .15, .25, .6, 1.3, 2.7, 4.05] * 1e-3 J  Eoff_data=[0, .0007, .0066, .033, .066, .17, .33, .83, 1.5; 0, .001, .01, .05, .1, .25, .5, 1.2, 2.2] * 1e-3 J  Eon_data_3D=[zeros(2, 9, 3)] J  Eoff_data_3D=[zeros(2, 9, 3)] J  Tj_loss=[298.15, 398.15] K  Iout_data_loss=[0, .1, 1, 5, 10, 20, 40, 70, 100] A  Vce_loss=[0, 150, 300] V  Eon_scalar=Eon_m J  Eoff_scalar=Eoff_m J  Voff=Voff_sw_loss_m V  Iout_scalar=Ion_sw_loss_m A  useCurrentFromPreviousCycle=true  useVoltageFromPreviousCycle=true  diodeModelType=ee.enum.converters.diodeModelType.pwl  diodeTableType=ee.enum.diode.tableType.IfMat  diode_ReverseIVType=ee.enum.diode.diodeReverseIV.constant  diode_IfMat=[.07, .12, .19, 1.75, 4.24, 7.32, 11.2; .16, .3, .72, 2.14, 4.02, 6.35, 9.12] A  diode_VfMat=[.9, 1.15, 1.25, 1.5, 1.75, 2.17, 2.6, 2.85; .58, .68, .75, 1.1, 1.38, 1.77, 2.27, 2.7] V  diode_TjVec=[25, 125] degC  diode_VfVec=[.5, .7, .9, 1.3, 1.7, 2.1, 2.5] V  diode_IfVec=[.1, .2, .5, 1, 2, 4, 7, 10] A  diode_IrMat=[1e-06, 2e-06, 5e-06, 1e-05, 2.5e-05, 5e-05, .0001; 2e-06, 5e-06, 1e-05, 4e-05, 8e-05, .0002, .0005] A  diode_VrMat=[10, 100, 200, 250, 300, 325, 350; 10, 70, 160, 220, 270, 300, 320] V  diode_VrVec=[10, 20, 40, 50, 70, 80, 100] V  diode_IrVec=[1e-06, 2e-06, 5e-06, 1e-05, 2e-05, 5e-05, .0001] A  diode_Vr=-600 V  diode_Ls=150 nH  diode_Erec=0.03 J  diode_rec_loss_model=ee.enum.diode.reverseRecoveryModel.fixed  diode_ErecVal=Erec_m J  diode_scaleWithIandV=true  diode_ErecMat=zeros(2, 3) J  diodeErecMat3D=zeros(2, 3, 2) J  diode_TjrecVec=[298.15, 398.15] K  diode_IfrecVec=[.1, 1, 10] A  diodeVrecVec=[0, 100] V  diode_IrecVal=Ion_sw_loss_m A  diode_VrecVal=Voff_sw_loss_m V  diode_tFilter=tc_m*100 s  separateThermalPortForDiode=false  thermal_network_parameterization=ee.enum.thermalNetworkTopology.external  Rth=[.08, .5] K/W  Rth_Cauer=[.08, .1, .5] K/W  Rth_Foster=[.08, .14, .22, .16] K/W  thermal_mass_parameterization=ee.enum.thermalNetwork.timeconstant  thermal_mass=[.01, .5] J/K  thermal_mass_Cauer=[.01, .1, .5] J/K  thermal_mass_Foster=[.001, .005, .05, .5] J/K  thermal_time_constant=[.001, .2] s  thermal_time_constant_Cauer=[.001, .1, .2] s  thermal_time_constant_Foster=[7e-05, .0007, .01, .08] s  thermal_mass_initial_temperatures=[25, 25] degC  thermal_mass_initial_temperatures_Cauer=[25, 25, 25] degC  junction_thermal_mass=JunctionTermalMass_m J/K  Tvec_initial_Foster=[25, 25, 25, 25] degC  RthDiode=[.03, .2] K/W  RthCauerDiode=[.03, .1, .2] K/W  RthFosterDiode=[.03, .2] K/W  thermalMassDiode=[3, 25] J/K  thermalMassCauerDiode=[3, 10, 25] J/K  thermalMassFosterDiode=[33, 50] J/K  thermalTauDiode=[.1, 5] s  thermalTauCauerDiode=[.1, 1, 5] s  thermalTauFosterDiode=[1, 10] s  thermalMassInitTempDiode=[25, 25] degC  thermalMassInitTempCauerDiode=[25, 25, 25] degC  junctionthermalMassDiode=0.1 J/K  TVecInitialFosterDiode=[25, 25, 25, 25] degC  no_thermal_network=0  IGBT_junction_temperature_specify=on  IGBT_junction_temperature_priority=High  IGBT_junction_temperature=Tambient_m degC  IGBT_junction_temperature_nominal_specify=off  IGBT_junction_temperature_nominal_value=1  IGBT_junction_temperature_nominal_unit=degC  diode_junction_temperature_specify=off  diode_junction_temperature_priority=None  diode_junction_temperature=25 degC  diode_junction_temperature_nominal_specify=off  diode_junction_temperature_nominal_value=1  diode_junction_temperature_nominal_unit=degC  Qj_specify=off  Qj_priority=None  Qj=0 W  Qj_nominal_specify=off  Qj_nominal_value=1  Qj_nominal_unit=W  accumulatedSwitchingLosses_specify=off  accumulatedSwitchingLosses_priority=None  accumulatedSwitchingLosses=0 J
  PS-Simulink Converter : nesl_utility/PS-Simulink Converter  PhysicalDomain=network_engine_domain  SubClassName=ps_output  LeftPortType=input  RightPortType=output  PseudoPeriodic=off  Frequencies=[]  VectorFormat=1-D array  Unit=W  AffineConversion=off
  PS-Simulink Converter{1..2,4..5} (4 alike) : nesl_utility/PS-Simulink Converter  PhysicalDomain=network_engine_domain  SubClassName=ps_output  LeftPortType=input  RightPortType=output  PseudoPeriodic=off  Frequencies=[]  VectorFormat=1-D array  Unit=degC  AffineConversion=off
  PS-Simulink Converter3 : nesl_utility/PS-Simulink Converter  PhysicalDomain=network_engine_domain  SubClassName=ps_output  LeftPortType=input  RightPortType=output  PseudoPeriodic=off  Frequencies=[]  VectorFormat=1-D array  Unit=W  AffineConversion=off
  Tambient : fl_lib/Thermal/Thermal Sources/Temperature Source  temperature=Tambient_m degC
  Temperature Sensor{,1..3} (4 alike) : fl_lib/Thermal/Thermal Sensors/Temperature Sensor  temperature_measure=foundation.enum.MeasurementReference.difference
  Voltage Sensor : fl_lib/Electrical/Electrical Sensors/Voltage Sensor
  diode_heatsink : fl_lib/Thermal/Thermal Elements/Thermal Resistance  resistance=rth_diode_HA_m K/W  T_specify=off  T_priority=High  T=0 deltadegC  T_nominal_specify=off  T_nominal_value=1  T_nominal_unit=K  Q_specify=off  Q_priority=None  Q=0 W  Q_nominal_specify=off  Q_nominal_value=1  Q_nominal_unit=W
  diode_sandwich : fl_lib/Thermal/Thermal Elements/Thermal Resistance  resistance=rth_diode_JH_m K/W  T_specify=off  T_priority=High  T=0 degC  T_nominal_specify=off  T_nominal_value=1  T_nominal_unit=K  Q_specify=off  Q_priority=None  Q=0 W  Q_nominal_specify=off  Q_nominal_value=1  Q_nominal_unit=W
  heatsink_C : fl_lib/Thermal/Thermal Elements/Thermal Mass  mass_type=foundation.enum.constant_variable.constant  mass=mass_heatsink_m kg  sp_heat=specific_heat_m J/(K*kg)  mass_min=1e-6 kg  num_ports=foundation.enum.numPorts2.one  m_specify=off  m_priority=High  m=1 kg  m_nominal_specify=off  m_nominal_value=1  m_nominal_unit=kg  T_specify=on  T_priority=High  T=DThs_init+Tambient degC  T_nominal_specify=off  T_nominal_value=1  T_nominal_unit=K  Q_specify=off  Q_priority=High  Q=0 W  Q_nominal_specify=off  Q_nominal_value=1  Q_nominal_unit=W
  heatsink_D : fl_lib/Thermal/Thermal Elements/Thermal Mass  mass_type=foundation.enum.constant_variable.constant  mass=mass_heatsink_m kg  sp_heat=specific_heat_m J/(K*kg)  mass_min=1e-6 kg  num_ports=foundation.enum.numPorts2.one  m_specify=off  m_priority=High  m=1 kg  m_nominal_specify=off  m_nominal_value=1  m_nominal_unit=kg  T_specify=on  T_priority=High  T=DThs_init+Tambient degC  T_nominal_specify=off  T_nominal_value=1  T_nominal_unit=K  Q_specify=off  Q_priority=High  Q=0 W  Q_nominal_specify=off  Q_nominal_value=1  Q_nominal_unit=W
  iph1 : nesl_utility/PS-Simulink Converter  PhysicalDomain=network_engine_domain  SubClassName=ps_output  LeftPortType=input  RightPortType=output  PseudoPeriodic=off  Frequencies=[]  VectorFormat=1-D array  Unit=A  AffineConversion=off
  power_losses_diode : fl_lib/Thermal/Thermal Sensors/Heat Flow Rate Sensor
  power_losses_switch : fl_lib/Thermal/Thermal Sensors/Heat Flow Rate Sensor
  switch_heatsink : fl_lib/Thermal/Thermal Elements/Thermal Resistance  resistance=rth_switch_HA_m K/W  T_specify=off  T_priority=High  T=0 deltadegC  T_nominal_specify=off  T_nominal_value=1  T_nominal_unit=K  Q_specify=off  Q_priority=None  Q=0 W  Q_nominal_specify=off  Q_nominal_value=1  Q_nominal_unit=W
  switch_sandwich : fl_lib/Thermal/Thermal Elements/Thermal Resistance  resistance=rth_switch_JH_m K/W  T_specify=off  T_priority=High  T=0 degC  T_nominal_specify=off  T_nominal_value=1  T_nominal_unit=K  Q_specify=off  Q_priority=None  Q=0 W  Q_nominal_specify=off  Q_nominal_value=1  Q_nominal_unit=W
  uph : nesl_utility/PS-Simulink Converter  PhysicalDomain=network_engine_domain  SubClassName=ps_output  LeftPortType=input  RightPortType=output  PseudoPeriodic=off  Frequencies=[]  VectorFormat=1-D array  Unit=V  AffineConversion=off
  G : PMIOPort  Side=Left
  C : PMIOPort  Port=2  Side=Left
  E : PMIOPort  Port=3  Side=Right
  tag scope: diode_HA_temp_Q1=scoped, diode_JH_temp_Q1=scoped, diode_ploss_Q1=scoped, igbt_HA_temp_Q1=scoped, igbt_JH_temp_Q1=scoped, igbt_current_Q1=scoped, igbt_ploss_Q1=scoped, igbt_voltage_Q1=scoped
  wires:
  PS-Simulink Converter/1 -> [igbt_ploss_Q1]  "Power Losses"
  PS-Simulink Converter2/1 -> [igbt_HA_temp_Q1]  "igbt_HA_temp"
  PS-Simulink Converter1/1 -> [igbt_JH_temp_Q1]  "igbt_JH_temp"
  iph1/1 -> [igbt_current_Q1]  "i_device_thermal_inv"
  uph/1 -> [igbt_voltage_Q1]  "uph"
  PS-Simulink Converter3/1 -> [diode_ploss_Q1]  "Power Losses"
  PS-Simulink Converter4/1 -> [diode_JH_temp_Q1]  "diode_JH_temp"
  PS-Simulink Converter5/1 -> [diode_HA_temp_Q1]  "diode_HA_temp"
  connections:
  Voltage Sensor/RConn2 -- Capacitor/RConn1 -- Diode/LConn1 -- "IGBT (Ideal, Switching)"/RConn2 -- E/RConn1
  "IGBT (Ideal, Switching)"/LConn1 -- G/RConn1
  PS-Simulink Converter/LConn1 -- power_losses_switch/RConn1
  Temperature Sensor/LConn1 -- power_losses_switch/RConn2 -- switch_sandwich/LConn1
  Temperature Sensor1/LConn1 -- Temperature Sensor/RConn1 -- switch_sandwich/RConn1 -- switch_heatsink/LConn1 -- heatsink_C/LConn1
  Temperature Sensor/RConn2 -- PS-Simulink Converter1/LConn1
  diode_heatsink/RConn1 -- Temperature Sensor2/RConn1 -- Temperature Sensor1/RConn1 -- Tambient/LConn1 -- switch_heatsink/RConn1
  Temperature Sensor1/RConn2 -- PS-Simulink Converter2/LConn1
  "IGBT (Ideal, Switching)"/LConn2 -- power_losses_switch/LConn1
  Current Sensor1/LConn1 -- C/RConn1
  Capacitor/LConn1 -- Voltage Sensor/LConn1 -- Diode/RConn1 -- Current Sensor1/RConn2 -- "IGBT (Ideal, Switching)"/RConn1
  Current Sensor1/RConn1 -- iph1/LConn1
  Voltage Sensor/RConn1 -- uph/LConn1
  Diode/LConn2 -- power_losses_diode/LConn1
  power_losses_diode/RConn2 -- Temperature Sensor3/LConn1 -- diode_sandwich/LConn1
  heatsink_D/LConn1 -- Temperature Sensor2/LConn1 -- Temperature Sensor3/RConn1 -- diode_sandwich/RConn1 -- diode_heatsink/LConn1
  power_losses_diode/RConn1 -- PS-Simulink Converter3/LConn1
  Temperature Sensor2/RConn2 -- PS-Simulink Converter5/LConn1
  Temperature Sensor3/RConn2 -- PS-Simulink Converter4/LConn1
